simulink model "ThreeOmniwheelMobileRobot"  (R2022a)
settings: Solver=VariableStepAuto  StartTime=0.0  StopTime=200  RelTol=1e-3
values from neighbouring files (symbols this model uses):
  ki = 0.015    [ParameterMobileRobot.m]
  kp = 0.02    [ParameterMobileRobot.m]
  kpx = 0.8    [ParameterMobileRobot.m]
  kpy = 0.8    [ParameterMobileRobot.m]
  ks = Km    (= 500)    [ParameterMobileRobot.m]
  L = 0.27    [ParameterMobileRobot.m]
  R = 0.06    [ParameterMobileRobot.m]
  tau = 2    [ParameterMobileRobot.m]
settings Model: Creator=84832  LastModifiedBy=lepha

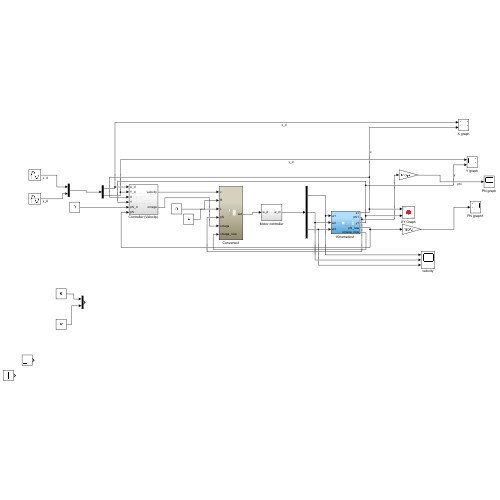
[thumbnail: Simulink's stored preview of the top-level diagram]
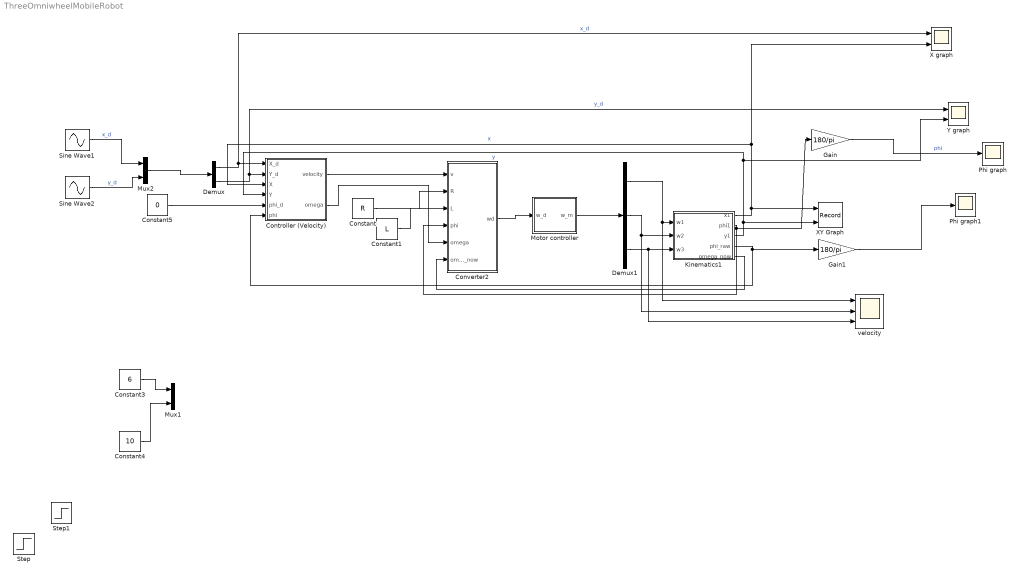
== system ThreeOmniwheelMobileRobot ==
  Constant : Constant  Value=R
  Constant1 : Constant  Value=L
  Constant3 : Constant  Value=6
  Constant4 : Constant  Value=10
  Constant5 : Constant  Value=0
  Controller (Velocity) : Subsystem
  Converter2 : Subsystem
  Demux : Demux  Outputs=2
  Demux1 : Demux  Outputs=3
  Gain : Gain  Gain=180/pi
  Gain1 : Gain  Gain=180/pi
  Kinematics1 : Subsystem
  Motor controller : Subsystem
  Mux1 : Mux  Inputs=2
  Mux2 : Mux  Inputs=2
  Phi graph : Scope
  Phi graph1 : Scope
  Sine Wave1 : Sin  Amplitude=5  Frequency=0.15  SampleTime=0
  Sine Wave2 : Sin  Amplitude=5  Frequency=0.15  Phase=pi/2  SampleTime=0
  Step : Step  After=2  SampleTime=0
  Step1 : Step  After=2  SampleTime=0
  X graph : Scope  NumInputPorts=2
  XY Graph : Record  FileSettingsInternal="{\"entries\":[{\"content\":{\"excelSettings\":{\"content\":{},\"type\":\"Streamout.ExcelSettings\"}},\"type\":\"Streamout.FileSettingStorage\",\"uuid\":\"f126f158-b8c3-4049-b826-cb05c3c9d9b4\"}],\"packageUris\":[\"http://schema.mathworks.com/mf0/streamout_blocks/R2020a\"],\"version\":\"1.0\"}"  Layout=[1 1]  SignalsInternal="{\"entries\":[{\"content\":{\"signals\":[{\"content\":{\"blockPath\":[\"new_test/XY Graph\"],\"channel\":[],\"dimensions\":[1],\"domain\":\"new_test/XY Graph\",\"lineColor\":\"#a2142f\",\"plots\":[1],\"port\":1,\"sid\":[\"\"],\"signalID\":9786,\"signalName\":\"x\"},\"type\":\"RecordBlkView.Signal\",\"uuid\":\"c76f9a00-786b-4790-a8b8-06553de90f4f\"},{\"content\":{\"blockPath\":[\"new_test/XY Graph\"],\"channel\":[],\"dimensions\":[1],\"domain\":\"new_test/XY Graph\",\"lineColor\":\"#139fff\",\"plots\":[1],\"port\":2,\"sid\":[\"\"],\"signalID\":9790,\"signalName\":\"y\"},\"type\":\"RecordBlkView.Signal\",\"uuid\":\"00e11548-94e1-48b9-9ce7-bb5dc2752333\"}]},\"type\":\"RecordBlkView.InputSignals\",\"uuid\":\"758b5c2c-26b4-4ce4-8a05-252aaf976e36\"}],\"packageUris\":[\"http://schema.mathworks.com/mf0/streamout_blocks/R2020a\"],\"version\":\"1.0\"}"  VisualizationBindings="{\"xyplotplugin\":{\"info\":[{\"series\":[{\"bindingParametersList\":[{\"parameter\":\"X-Axis\",\"signalID\":9786,\"signalName\":\"x\"},{\"parameter\":\"Y-Axis\",\"signalID\":9790,\"signalName\":\"y\"}],\"seriesID\":123}],\"subplotID\":1}]}}"  CompatibilityTag=XY
  Y graph : Scope  NumInputPorts=2
  velocity : Scope  NumInputPorts=3
  wires:
  Demux/1 -> X graph/1, Controller (Velocity)/1(X_d)  "x_d"
  Demux/2 -> Y graph/1, Controller (Velocity)/2(Y_d)  "y_d"
  Constant/1 -> Converter2/2(R)
  Constant1/1 -> Converter2/3(L)
  Motor controller/1(w_m) -> Demux1/1
  Kinematics1/1(x1) -> X graph/2, Controller (Velocity)/3(X), XY Graph/1  "x"
  Kinematics1/3(y1) -> Y graph/2, Controller (Velocity)/4(Y), XY Graph/2  "y"
  Kinematics1/2(phi1) -> Converter2/4(phi), Gain/1
  Gain/1 -> Phi graph/1  "phi"
  Demux1/1 -> velocity/1, Kinematics1/1(w1)
  Demux1/2 -> velocity/2, Kinematics1/2(w2)
  Sine Wave1/1 -> Mux2/1  "x_d"
  Sine Wave2/1 -> Mux2/2  "y_d"
  Converter2/1(wd) -> Motor controller/1(w_d)
  Demux1/3 -> Kinematics1/3(w3), velocity/3
  Controller (Velocity)/1(velocity) -> Converter2/1(v)
  Controller (Velocity)/2(omega) -> Converter2/5(omega)
  Constant3/1 -> Mux1/1
  Constant4/1 -> Mux1/2
  Constant5/1 -> Controller (Velocity)/5(phi_d)
  Kinematics1/4(phi_raw) -> Gain1/1, Controller (Velocity)/6(phi)
  Gain1/1 -> Phi graph1/1
  Kinematics1/5(omega_now) -> Converter2/6(omega_now)
  Mux2/1 -> Demux/1

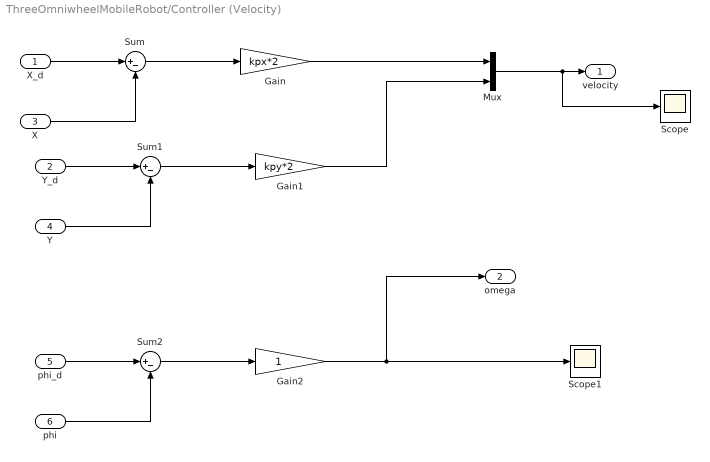
== system ThreeOmniwheelMobileRobot/Controller (Velocity) ==
  X_d : Inport
  Y_d : Inport  Port=2
  X : Inport  Port=3
  Y : Inport  Port=4
  phi_d : Inport  Port=5
  phi : Inport  Port=6
  Gain : Gain  Gain=kpx*2
  Gain1 : Gain  Gain=kpy*2
  Gain2 : Gain
  Mux : Mux  Inputs=2
  Scope : Scope
  Scope1 : Scope
  Sum : Sum  Inputs=|+-
  Sum1 : Sum  Inputs=|+-
  Sum2 : Sum  Inputs=|+-
  velocity : Outport
  omega : Outport  Port=2
  wires:
  Y_d/1 -> Sum1/1
  X_d/1 -> Sum/1
  Gain1/1 -> Mux/2
  Gain/1 -> Mux/1
  Y/1 -> Sum1/2
  X/1 -> Sum/2
  Sum1/1 -> Gain1/1
  Sum/1 -> Gain/1
  Mux/1 -> Scope/1, velocity/1
  phi/1 -> Sum2/2
  phi_d/1 -> Sum2/1
  Sum2/1 -> Gain2/1
  Gain2/1 -> Scope1/1, omega/1

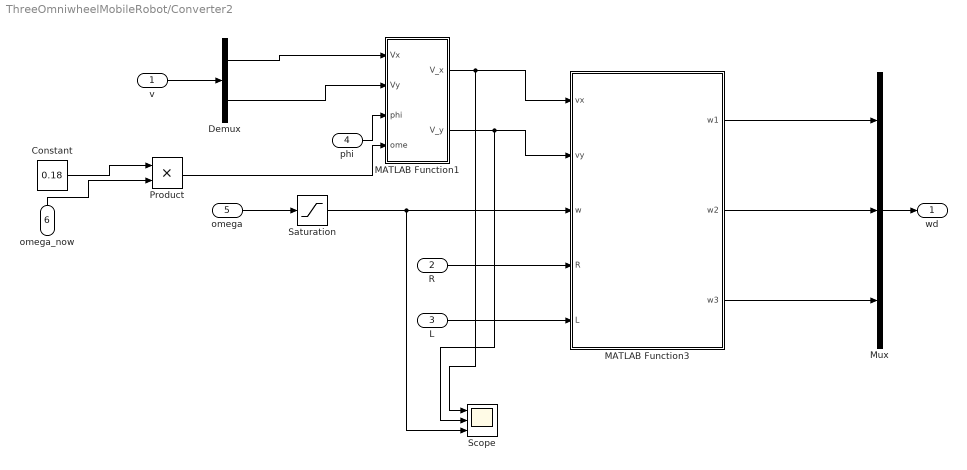
== system ThreeOmniwheelMobileRobot/Converter2 ==
  v : Inport
  R : Inport  Port=2
  L : Inport  Port=3
  phi : Inport  Port=4
  omega : Inport  Port=5
  omega_now : Inport  Port=6
  Constant : Constant  Value=0.18
  Demux : Demux  Outputs=2
  MATLAB Function1 : MATLAB Function  TreatAsAtomicUnit=on
  MATLAB Function3 : MATLAB Function  TreatAsAtomicUnit=on
  Mux : Mux  Inputs=3
  Product : Product
  Saturation : Saturate  UpperLimit=10
  Scope : Scope  NumInputPorts=3
  wd : Outport
  wires:
  L/1 -> MATLAB Function3/5(L)
  R/1 -> MATLAB Function3/4(R)
  phi/1 -> MATLAB Function1/3(phi)
  MATLAB Function1/1(V_x) -> Scope/1, MATLAB Function3/1(vx)
  MATLAB Function1/2(V_y) -> Scope/2, MATLAB Function3/2(vy)
  MATLAB Function3/1(w1) -> Mux/1
  MATLAB Function3/2(w2) -> Mux/2
  MATLAB Function3/3(w3) -> Mux/3
  Mux/1 -> wd/1
  v/1 -> Demux/1
  Demux/1 -> MATLAB Function1/1(Vx)
  Demux/2 -> MATLAB Function1/2(Vy)
  omega/1 -> Saturation/1
  Product/1 -> MATLAB Function1/4(ome)
  Constant/1 -> Product/1
  Saturation/1 -> Scope/3, MATLAB Function3/3(w)
  omega_now/1 -> Product/2

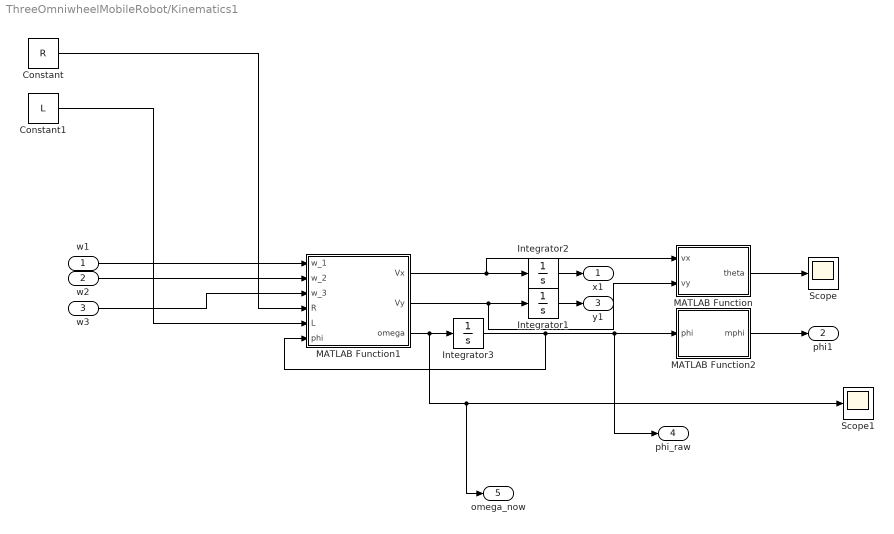
== system ThreeOmniwheelMobileRobot/Kinematics1 ==
  w1 : Inport
  w2 : Inport  Port=2
  w3 : Inport  Port=3
  Constant : Constant  Value=R
  Constant1 : Constant  Value=L
  Integrator1 : Integrator
  Integrator2 : Integrator
  Integrator3 : Integrator
  MATLAB Function : MATLAB Function  TreatAsAtomicUnit=on
  MATLAB Function1 : MATLAB Function  TreatAsAtomicUnit=on
  MATLAB Function2 : MATLAB Function  TreatAsAtomicUnit=on
  Scope : Scope
  Scope1 : Scope
  x1 : Outport
  phi1 : Outport  Port=2
  y1 : Outport  Port=3
  phi_raw : Outport  Port=4
  omega_now : Outport  Port=5
  wires:
  w1/1 -> MATLAB Function1/1(w_1)
  w2/1 -> MATLAB Function1/2(w_2)
  Constant/1 -> MATLAB Function1/4(R)
  Constant1/1 -> MATLAB Function1/5(L)
  MATLAB Function1/3(omega) -> omega_now/1, Scope1/1, Integrator3/1
  Integrator3/1 -> phi_raw/1, MATLAB Function2/1(phi), MATLAB Function1/6(phi)
  MATLAB Function2/1(mphi) -> phi1/1
  MATLAB Function1/2(Vy) -> MATLAB Function/2(vy), Integrator1/1
  MATLAB Function1/1(Vx) -> MATLAB Function/1(vx), Integrator2/1
  w3/1 -> MATLAB Function1/3(w_3)
  MATLAB Function/1(theta) -> Scope/1
  Integrator1/1 -> y1/1
  Integrator2/1 -> x1/1

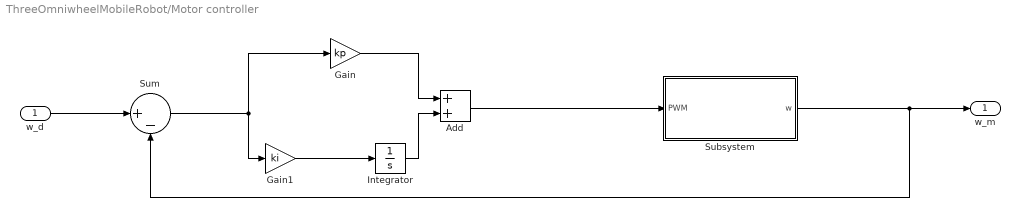
== system ThreeOmniwheelMobileRobot/Motor controller ==
  w_d : Inport
  Add : Sum
  Gain : Gain  Gain=kp
  Gain1 : Gain  Gain=ki
  Integrator : Integrator
  Subsystem : Subsystem
  Sum : Sum  Inputs=|+-
  w_m : Outport
  wires:
  w_d/1 -> Sum/1
  Add/1 -> Subsystem/1(PWM)
  Sum/1 -> Gain1/1, Gain/1
  Gain1/1 -> Integrator/1
  Subsystem/1(w) -> w_m/1, Sum/2
  Gain/1 -> Add/1
  Integrator/1 -> Add/2

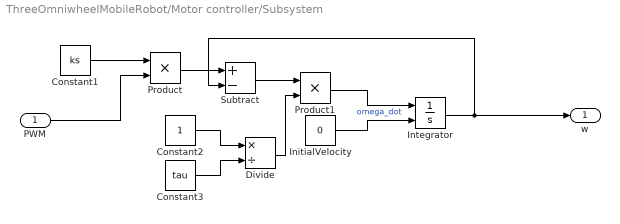
== system ThreeOmniwheelMobileRobot/Motor controller/Subsystem ==
  PWM : Inport
  Constant1 : Constant  Value=ks
  Constant2 : Constant
  Constant3 : Constant  Value=tau
  Divide : Product  Inputs=*/
  InitialVelocity : Constant  Value=0
  Integrator : Integrator  InitialConditionSource=external
  Product : Product
  Product1 : Product
  Subtract : Sum  Inputs=+-
  w : Outport
  wires:
  PWM/1 -> Product/2
  Product/1 -> Subtract/1
  Integrator/1 -> w/1, Subtract/2
  Constant2/1 -> Divide/1
  Product1/1 -> Integrator/1  "omega_dot"
  InitialVelocity/1 -> Integrator/2
  Divide/1 -> Product1/2
  Subtract/1 -> Product1/1
  Constant3/1 -> Divide/2
  Constant1/1 -> Product/1

== matlab function ThreeOmniwheelMobileRobot/Kinematics1/MATLAB Function1 ==
  data: w_1 input; Vx output; w_2 input; w_3 input; R input; L input; Vy output; omega output; phi input
function [Vx,Vy,omega] = fcn(w_1, w_2, w_3, R,L, phi)
matrixV = R*[w_1;w_2;w_3];
cvert = [0 -(sqrt(3)/3) (sqrt(3)/3);
    2/3 -1/3 -1/3 ;
    1/3*L 1/3*L 1/3*L];


a = cvert*matrixV;
b=[cos(phi) -sin(phi) 0; sin(phi) cos(phi) 0; 0 0 1]*[a(1);a(2);0];
Vx = b(1);
Vy = b(2);
omega = a(3);

== matlab function ThreeOmniwheelMobileRobot/Kinematics1/MATLAB Function2 ==
  data: phi input; mphi output
function mphi = fcn(phi)

rphi=mod(phi,2*pi);

if rphi<=-pi
    mphi=rphi+2*pi;
elseif rphi>pi
    mphi=rphi-2*pi;
else
    mphi=rphi;
end

== matlab function ThreeOmniwheelMobileRobot/Kinematics1/MATLAB Function ==
  data: vx input; theta output; vy input
function theta = fcn(vx,vy)

theta = atan2(vy,vx);

== matlab function ThreeOmniwheelMobileRobot/Converter2/MATLAB Function1 ==
  data: Vx input; V_x output; Vy input; phi input; V_y output; ome input
function [V_x,V_y] = fcn(Vx,Vy,phi,ome)
matrixV = [Vx;Vy;0];
a= [cos(-phi) -sin(-phi) 0; sin(-phi) cos(-phi) 0; 0 0 1]*matrixV;


V_x = a(1) + ome*a(2);
V_y = a(2) - ome*a(1);

== matlab function ThreeOmniwheelMobileRobot/Converter2/MATLAB Function3 ==
  data: vx input; w1 output; vy input; w input; w2 output; w3 output; R input; L input
function [w1,w2,w3] = fcn(vx,vy,w,R,L)
invMatrix = [0 1 1/L;
    -3^(1/2)/2 -1/2 1/L;
     3^(1/2)/2 -1/2 1/L];
a= [vx;vy;w];
b= invMatrix*a;

w1 = b(1)/R;
w2 = b(2)/R;
w3 = b(3)/R;
